simulink model "SingleInverterSim"  (R2020b)
settings: Solver=FixedStepAuto  StartTime=0.0  StopTime=3  FixedStep=Ts  RelTol=1e-3
values from neighbouring files (symbols this model uses):
  Cf = 0.02/W    (= 6.36619772368e-05)    [CalcSwingDroop.m]    (also in SingleInverterSim_Para.m = 0.02; SingleInverterSim_Para_v2.m = 0.02)
  Lc = 0.01/W    (= 3.18309886184e-05)    [CalcSwingDroop.m]    (also in SingleInverterSim_Para.m = 1e-09; SingleInverterSim_Para_v2.m = 0.01)
  Lf = 0.05/W    (= 0.000159154943092)    [CalcSwingDroop.m]    (also in SingleInverterSim_Para.m = 0.05; SingleInverterSim_Para_v2.m = 0.05)
  m = m*Wbase    (= 15.7079632679)    [CalcSwingDroop.m]    (also in SingleInverterSim_Para.m = 0.05; SingleInverterSim_Para_v2.m = 0.05)
  R_rated_GFL = X_rated_GFL/5    (= 0.08)    [SingleInverterSim_Para.m]
  R_rated_GFM = X_rated_GFM/5    (= 0.06)    [SingleInverterSim_Para.m]
  Sbase = 1    [MainAnalysisImpedanceCircuit.m]    (also in SingleInverterSim_Para.m; SingleInverterSim_Para_v2.m)
  Scale_ki_v = 20    [SingleInverterSim_Para.m]    (also in SingleInverterSim_Para_v2.m)
  Ts = 1/Fs    (= 0.0001)    [SingleInverterSim_Para.m]    (also in SingleInverterSim_Para_v2.m)
  Vbase = 1    [MainAnalysisImpedanceCircuit.m]    (also in SingleInverterSim_Para.m; SingleInverterSim_Para_v2.m)
  w_droop = 0.1*2*pi    (= 0.628318530718)    [SingleInverterSim_Para.m]    (also in SingleInverterSim_Para_v2.m = 62.8318530718)
  w_i_GFL = 250 *2*pi    (= 1570.79632679)    [SingleInverterSim_Para.m]    (also in SingleInverterSim_Para_v2.m = 3141.59265359)
  w_i_GFM = 500*2*pi    (= 3141.59265359)    [SingleInverterSim_Para.m]    (also in SingleInverterSim_Para_v2.m)
  w_pll = 15 *2*pi    (= 94.2477796077)    [SingleInverterSim_Para.m]    (also in SingleInverterSim_Para_v2.m = 62.8318530718)
  w_tau = 1e3 *2*pi    (= 6283.18530718)    [SingleInverterSim_Para.m]    (also in SingleInverterSim_Para_v2.m)
  w_v_GFM = 250 *2*pi    (= 1570.79632679)    [SingleInverterSim_Para.m]    (also in SingleInverterSim_Para_v2.m)
  Wbase = 2*pi*50    (= 314.159265359)    [CalcSwingDroop.m]    (also in MainAnalysisImpedanceCircuit.m; SingleInverterSim_Para.m; SingleInverterSim_Para_v2.m)
  X_rated_GFL = 0.4    [SingleInverterSim_Para.m]
  X_rated_GFM = 0.3    [SingleInverterSim_Para.m]
  Zbase = Vbase/Ibase    (= 1)    [MainAnalysisImpedanceCircuit.m]    (also in SingleInverterSim_Para.m; SingleInverterSim_Para_v2.m)
undefined symbols (not defined in the file or in its folder): DiscIntNeverNeededParam, initial, magnitude
libraries: powerlib x230, SimplexPS x57, SimplexPS_2015a x10, SimplusGT x3
(part 1 of 5)
settings Model: Creator=admin_user  LastModifiedBy=admin_user
settings DataIOCC: SaveOutput=off  SignalLogging=off  DSMLogging=off  SaveTime=off  ReturnWorkspaceOutputs=off

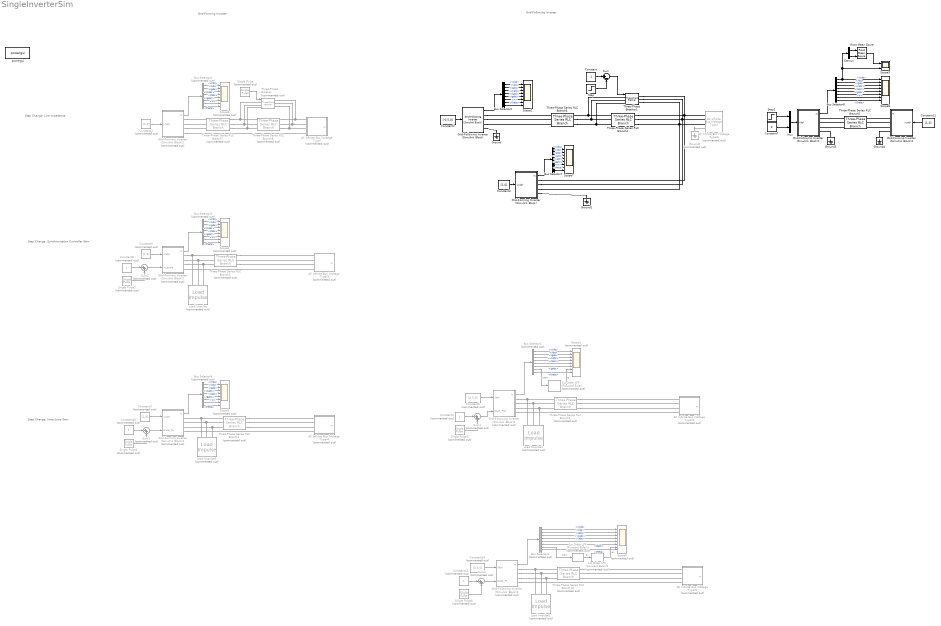
== system SingleInverterSim ==
  note: Step Change:
      | Line Impedance
  note: Grid-Forming Inverter
  note: Grid-Following Inverter
  note: Step Change:
      | Synchronization Controller Gain
  note: Step Change:
      | Inner-Loop Gain
  1st Order LPF (Forward Euler) : SimplexPS/1st Order LPF (Forward Euler)  Commented=on  wc=100*2*pi  Ts=Ts
      settings: SourceProductName=Simplex Power Systems
  1st Order LPF (Forward Euler)1 : SimplexPS/1st Order LPF (Forward Euler)  Commented=on  wc=100*2*pi  Ts=Ts
      settings: SourceProductName=Simplex Power Systems
  1st Order LPF (Forward Euler)2 : SimplexPS/1st Order LPF (Forward Euler)  Commented=on  wc=100*2*pi  Ts=Ts
      settings: SourceProductName=Simplex Power Systems
  AC Infinite Bus (Voltage Type) : Subsystem  Commented=on  AncestorBlock=|  mask{Ts=Ts, Sbase=Sbase, Vbase=Vbase, Wbase=Wbase, vd=1, vq=0, theta0=0, w=Wbase, R=1e-30}
      | SimplexPS/AC Infinite Bus
      | (Voltage Type)
      mask prompts: Ts "Ts (s), samping period"; Sbase "Sbase (VA), power base"; Vbase "Vbase (V), voltage base"; Wbase "Wbase (rad/s), frequency base"; vd "vd (pu), d-axis voltage"; vq "vq (pu), q-axis voltage"; theta0 "theta0 (rad), initial angle"; w "w (rad/s), frequency"; R "R (Ohm), resistance"
  AC Infinite Bus (Voltage Type)2 : Subsystem  Commented=on  AncestorBlock=|  mask{Ts=Ts, Sbase=Sbase, Vbase=Vbase, Wbase=Wbase, vd=1, vq=0, theta0=0, w=Wbase, R=1e-30}
      | SimplexPS/AC Infinite Bus
      | (Voltage Type)
      mask prompts: Ts "Ts (s), samping period"; Sbase "Sbase (VA), power base"; Vbase "Vbase (V), voltage base"; Wbase "Wbase (rad/s), frequency base"; vd "vd (pu), d-axis voltage"; vq "vq (pu), q-axis voltage"; theta0 "theta0 (rad), initial angle"; w "w (rad/s), frequency"; R "R (Ohm), resistance"
  AC Infinite Bus (Voltage Type)3 : Subsystem  Commented=on  AncestorBlock=|  mask{Ts=Ts, Sbase=Sbase, Vbase=Vbase, Wbase=Wbase, vd=1, vq=0, theta0=0, w=Wbase, R=1e-30}
      | SimplexPS/AC Infinite Bus
      | (Voltage Type)
      mask prompts: Ts "Ts (s), samping period"; Sbase "Sbase (VA), power base"; Vbase "Vbase (V), voltage base"; Wbase "Wbase (rad/s), frequency base"; vd "vd (pu), d-axis voltage"; vq "vq (pu), q-axis voltage"; theta0 "theta0 (rad), initial angle"; w "w (rad/s), frequency"; R "R (Ohm), resistance"
  AC Infinite Bus (Voltage Type)4 : Subsystem  Commented=on  AncestorBlock=|  mask{Ts=Ts, Sbase=Sbase, Vbase=Vbase, Wbase=Wbase, vd=1, vq=0, theta0=0, w=Wbase, R=1e-30}
      | SimplexPS/AC Infinite Bus
      | (Voltage Type)
      mask prompts: Ts "Ts (s), samping period"; Sbase "Sbase (VA), power base"; Vbase "Vbase (V), voltage base"; Wbase "Wbase (rad/s), frequency base"; vd "vd (pu), d-axis voltage"; vq "vq (pu), q-axis voltage"; theta0 "theta0 (rad), initial angle"; w "w (rad/s), frequency"; R "R (Ohm), resistance"
  AC Infinite Bus (Voltage Type)5 : Subsystem  Commented=on  AncestorBlock=|  mask{Ts=Ts, Sbase=Sbase, Vbase=Vbase, Wbase=Wbase, vd=1, vq=0, theta0=0, w=Wbase, R=1e-30}
      | SimplexPS/AC Infinite Bus
      | (Voltage Type)
      mask prompts: Ts "Ts (s), samping period"; Sbase "Sbase (VA), power base"; Vbase "Vbase (V), voltage base"; Wbase "Wbase (rad/s), frequency base"; vd "vd (pu), d-axis voltage"; vq "vq (pu), q-axis voltage"; theta0 "theta0 (rad), initial angle"; w "w (rad/s), frequency"; R "R (Ohm), resistance"
  AC Infinite Bus (Voltage Type)6 : SimplusGT/AC Infinite Bus (Voltage Type)  Commented=on  Ts=Ts  Sbase=Sbase  Vbase=Vbase  Wbase=Wbase  vd=1  vq=0  theta0=0  w=Wbase  R=1e-30
      settings: SourceProductName=Simplus Grid Tool
  Bus Selector{1,3..6} (5 alike) : BusSelector  Commented=on  OutputSignals=vcdq,ildq,igdq,vcabc,ilabc,igabc,w,theta
  Bus Selector2 : BusSelector  OutputSignals=vcdq,ildq,igdq,vcabc,ilabc,igabc,w,theta
  Bus Selector7 : BusSelector  OutputSignals=vcdq,ildq,igdq,vcabc,ilabc,igabc,w,theta
  Bus Selector8 : BusSelector  OutputSignals=vcdq,ildq,igdq,vcabc,ilabc,igabc,w,theta
  Constant : Constant
  Constant1 : Constant  Commented=on  Value=[1,0]
  Constant{4,8,10,13} (4 alike) : Constant  Commented=on
  Constant11 : Constant  Value=[1,0]
  Constant14 : Constant  Commented=on  Value=[0.5,0]
  Constant2 : Constant  Value=[-0.5,0]
  Constant3 : Constant  Value=[1,0]
  Constant5 : Constant  Commented=on  Value=[1,0]
  Constant6 : Constant  Commented=on  Value=[0.5,0]
  Constant7 : Constant  Value=0
  Constant9 : Constant  Commented=on  Value=[1,0]
  Demux : Demux  Outputs=2
  Grid-Following Inverter (Simulink Block) : SimplusGT/Grid-Following Inverter (Simulink Block)  Ts=Ts  Sbase=Sbase  Vbase=Vbase  Wbase=Wbase  w_i=w_i_GFL  w_pll=w_pll  w_tau=w_tau  Lf=Lf  Cf=Cf  Lc=Lc
      settings: SourceProductName=Simplus Grid Tool
  Grid-Following Inverter (Simulink Block)1 : Subsystem  AncestorBlock=|  mask{Ts=Ts, Sbase=Sbase, Vbase=Vbase, Wbase=Wbase, w_i=w_i_GFL, w_pll=w_pll/10, w_tau=w_tau, Lf=Lf, Cf=Cf, Lc=Lc}
      | SimplusGT/Grid-Following Inverter
      | (Simulink Block)
      mask prompts: Ts "Ts (s), sampling period"; Sbase "Sbase (VA), base power"; Vbase "Vbase (V), base voltage"; Wbase "Wbase (rad/s), base frequency"; w_i "w_i (rad/s), current-loop bandwidth"; w_pll "w_pll (rad/s), PLL bandwidth"; w_tau "w_tau (rad/s), PLL filter bandwidth"; Lf "Lf (pu), LCL filter"; Cf "Cf (pu), LCL filter"; Lc "Lc (pu), LCL filter"
  Grid-Following Inverter (Simulink Block)2 : Subsystem  Commented=on  AncestorBlock=|  mask{Ts=Ts, Sbase=Sbase, Vbase=Vbase, Wbase=Wbase, w_i=w_i_GFL, w_pll=w_pll, w_tau=w_tau, Lf=Lf, Cf=Cf, Lc=Lc}
      | SimplexPS/Grid-Following Inverter
      | (Simulink Block)
      mask prompts: Ts "Ts (s), sampling period"; Sbase "Sbase (VA), base power"; Vbase "Vbase (V), base voltage"; Wbase "Wbase (rad/s), base frequency"; w_i "w_i (rad/s), current-loop bandwidth"; w_pll "w_pll (rad/s), PLL bandwidth"; w_tau "w_tau (rad/s), PLL filter bandwidth"; Lf "Lf (pu), LCL filter"; Cf "Cf (pu), LCL filter"; Lc "Lc (pu), LCL filter"
  Grid-Following Inverter (Simulink Block)3 : Subsystem  Commented=on  AncestorBlock=|  mask{Ts=Ts, Sbase=Sbase, Vbase=Vbase, Wbase=Wbase, w_i=w_i_GFL, w_pll=w_pll, w_tau=w_tau, Lf=Lf, Cf=Cf, Lc=Lc}
      | SimplexPS/Grid-Following Inverter
      | (Simulink Block)
      mask prompts: Ts "Ts (s), sampling period"; Sbase "Sbase (VA), base power"; Vbase "Vbase (V), base voltage"; Wbase "Wbase (rad/s), base frequency"; w_i "w_i (rad/s), current-loop bandwidth"; w_pll "w_pll (rad/s), PLL bandwidth"; w_tau "w_tau (rad/s), PLL filter bandwidth"; Lf "Lf (pu), LCL filter"; Cf "Cf (pu), LCL filter"; Lc "Lc (pu), LCL filter"
  Grid-Forming Inverter (Simulink Block) : Subsystem  AncestorBlock=|  mask{Ts=Ts, Sbase=Sbase, Vbase=Vbase, Wbase=Wbase, w_i=w_i_GFM, w_v=w_v_GFM, w_droop=w_droop, m=m, Lf=Lf, Cf=Cf, Lc=Lc}
      | SimplusGT/Grid-Forming Inverter
      | (Simulink Block)
      mask prompts: Ts "Ts (s), sampling period"; Sbase "Sbase (VA), base power"; Vbase "Vbase (V), base voltage"; Wbase "Wbase (rad/s), base frequency"; w_i "w_i (rad/s), current-loop bandwidth"; w_v "w_v (rad/s), voltage-loop bandwidth"; w_droop "w_droop (rad/s), droop bandwidth"; m "m (pu), frequency droop gain"; Lf "Lf (pu), LCL filter"; Cf "Cf (pu), LCL filter"; Lc "Lc (pu), LCL filter"
  Grid-Forming Inverter (Simulink Block)1 : Subsystem  Commented=on  AncestorBlock=|  mask{Ts=Ts, Sbase=Sbase, Vbase=Vbase, Wbase=Wbase, w_i=w_i_GFM, w_v=w_v_GFM, w_droop=w_droop, m=m, Lf=Lf, Cf=Cf, Lc=Lc}
      | SimplexPS/Grid-Forming Inverter
      | (Simulink Block)
      mask prompts: Ts "Ts (s), sampling period"; Sbase "Sbase (VA), base power"; Vbase "Vbase (V), base voltage"; Wbase "Wbase (rad/s), base frequency"; w_i "w_i (rad/s), current-loop bandwidth"; w_v "w_v (rad/s), voltage-loop bandwidth"; w_droop "w_droop (rad/s), droop bandwidth"; m "m (pu), frequency droop gain"; Lf "Lf (pu), LCL filter"; Cf "Cf (pu), LCL filter"; Lc "Lc (pu), LCL filter"
  Grid-Forming Inverter (Simulink Block)2 : Subsystem  Commented=on  AncestorBlock=|  mask{Ts=Ts, Sbase=Sbase, Vbase=Vbase, Wbase=Wbase, w_i=w_i_GFM, w_v=w_v_GFM, w_droop=w_droop, m=m, Lf=Lf, Cf=Cf, Lc=Lc, Scale_ki_v=Scale_ki_v}
      | SimplexPS/Grid-Forming Inverter
      | (Simulink Block)
      mask prompts: Ts "Ts (s), sampling period"; Sbase "Sbase (VA), base power"; Vbase "Vbase (V), base voltage"; Wbase "Wbase (rad/s), base frequency"; w_i "w_i (rad/s), current-loop bandwidth"; w_v "w_v (rad/s), voltage-loop bandwidth"; w_droop "w_droop (rad/s), droop bandwidth"; m "m (pu), frequency droop gain"; Lf "Lf (pu), LCL filter"; Cf "Cf (pu), LCL filter"; Lc "Lc (pu), LCL filter"
  Grid-Forming Inverter (Simulink Block)3 : Subsystem  Commented=on  AncestorBlock=|  mask{Ts=Ts, Sbase=Sbase, Vbase=Vbase, Wbase=Wbase, w_i=w_i_GFM, w_v=w_v_GFM, w_droop=w_droop, m=m, Lf=Lf, Cf=Cf, Lc=Lc, Scale_ki_v=Scale_ki_v}
      | SimplexPS/Grid-Forming Inverter
      | (Simulink Block)
      mask prompts: Ts "Ts (s), sampling period"; Sbase "Sbase (VA), base power"; Vbase "Vbase (V), base voltage"; Wbase "Wbase (rad/s), base frequency"; w_i "w_i (rad/s), current-loop bandwidth"; w_v "w_v (rad/s), voltage-loop bandwidth"; w_droop "w_droop (rad/s), droop bandwidth"; m "m (pu), frequency droop gain"; Lf "Lf (pu), LCL filter"; Cf "Cf (pu), LCL filter"; Lc "Lc (pu), LCL filter"
  Grid-Forming Inverter (Simulink Block)4 : Subsystem  AncestorBlock=|  mask{Ts=Ts, Sbase=Sbase, Vbase=Vbase, Wbase=Wbase, w_i=w_i_GFM, w_v=w_v_GFM, w_droop=w_droop*100, m=m, Lf=Lf, Cf=Cf, Lc=Lc}
      | SimplusGT/Grid-Forming Inverter
      | (Simulink Block)
      mask prompts: Ts "Ts (s), sampling period"; Sbase "Sbase (VA), base power"; Vbase "Vbase (V), base voltage"; Wbase "Wbase (rad/s), base frequency"; w_i "w_i (rad/s), current-loop bandwidth"; w_v "w_v (rad/s), voltage-loop bandwidth"; w_droop "w_droop (rad/s), droop bandwidth"; m "m (pu), frequency droop gain"; Lf "Lf (pu), LCL filter"; Cf "Cf (pu), LCL filter"; Lc "Lc (pu), LCL filter"
  Ground{,1,3..4} (4 alike) : powerlib/Elements/Ground  LConnTagsString=a
  Ground2 : powerlib/Elements/Ground  Commented=on  LConnTagsString=a
  Load Impulse{,1..3} (4 alike) : SimplexPS/Load Impulse  Commented=on  t0=t0  dt=Ts  R=10000*Zbase
      settings: SourceProductName=Simplex Power Systems
  Mux : Mux  Inputs=2
  Root Mean Squre : SimplusGT/Root Mean Squre  SystemSampleTime=-1  VariantActivationTime=update diagram  Latency=0  AutoFrameSizeCalculation=off
      settings: SourceProductName=Simplus Grid Tool
  Scope{1,3..6} (5 alike) : Scope  Commented=on  NumInputPorts=8
  Scope2 : Scope  NumInputPorts=8
  Scope7 : Scope  NumInputPorts=8
  Scope8 : Scope  NumInputPorts=8
  Scope9 : Scope  NumInputPorts=2
  Single Pulse : SimplexPS/Single Pulse  Commented=on  t0=t0  dt=dt  Am=1
      settings: SourceProductName=Simplex Power Systems
  Single Pulse2 : SimplexPS/Single Pulse  Commented=on  t0=t0  dt=dt  Am=3
      settings: SourceProductName=Simplex Power Systems
  Single Pulse3 : SimplexPS/Single Pulse  Commented=on  t0=2  dt=0.2  Am=3
      settings: SourceProductName=Simplex Power Systems
  Single Pulse4 : SimplexPS/Single Pulse  Commented=on  t0=t0  dt=dt  Am=-2/5
      settings: SourceProductName=Simplex Power Systems
  Single Pulse5 : SimplexPS/Single Pulse  Commented=on  t0=t0  dt=dt  Am=-2/5
      settings: SourceProductName=Simplex Power Systems
  Step : Step  SampleTime=0
  Step1 : Step  After=0.5  SampleTime=0
  Sum : Sum  Inputs=|+-
  Sum{1..4} (4 alike) : Sum  Commented=on  Inputs=|++
  Three-Phase Series RLC Branch1 : powerlib/Elements/Three-Phase Series RLC Branch  Commented=on  LConnTagsString=A|B|C  RConnTagsString=A|B|C  BranchType=RL  Resistance=R_rated_GFM*Zbase  Inductance=X_rated_GFM*Zbase/Wbase  Capacitance=1/Wbase  Measurements=None
  Three-Phase Series RLC Branch10 : powerlib/Elements/Three-Phase Series RLC Branch  Commented=on  LConnTagsString=A|B|C  RConnTagsString=A|B|C  BranchType=RL  Resistance=R_rated_GFL*Zbase  Inductance=X_rated_GFL*Zbase/Wbase  Capacitance=1/Wbase  Measurements=None
  Three-Phase Series RLC Branch2 : powerlib/Elements/Three-Phase Series RLC Branch  Commented=on  LConnTagsString=A|B|C  RConnTagsString=A|B|C  BranchType=RL  Resistance=R_rated_GFL*Zbase  Inductance=X_rated_GFL*Zbase/Wbase  Capacitance=1/Wbase  Measurements=None
  Three-Phase Series RLC Branch3 : powerlib/Elements/Three-Phase Series RLC Branch  Commented=on  LConnTagsString=A|B|C  RConnTagsString=A|B|C  BranchType=RL  Resistance=R_rated_GFM*Zbase  Inductance=X_rated_GFM*Zbase/Wbase  Capacitance=1/Wbase  Measurements=None
  Three-Phase Series RLC Branch4 : powerlib/Elements/Three-Phase Series RLC Branch  LConnTagsString=A|B|C  RConnTagsString=A|B|C  BranchType=RL  Resistance=0.23*Zbase/10  Inductance=0.23*Zbase/Wbase  Capacitance=1/Wbase  Measurements=None
  Three-Phase Series RLC Branch5 : powerlib/Elements/Three-Phase Series RLC Branch  LConnTagsString=A|B|C  RConnTagsString=A|B|C  BranchType=RL  Resistance=0.1*Zbase/10  Inductance=0.1*Zbase/Wbase  Capacitance=1/Wbase  Measurements=None
  Three-Phase Series RLC Branch6 : powerlib/Elements/Three-Phase Series RLC Branch  LConnTagsString=A|B|C  RConnTagsString=A|B|C  BranchType=RL  Resistance=0.3*Zbase/10  Inductance=0.3*Zbase/Wbase  Capacitance=1/Wbase  Measurements=None
  Three-Phase Series RLC Branch7 : powerlib/Elements/Three-Phase Series RLC Branch  Commented=on  LConnTagsString=A|B|C  RConnTagsString=A|B|C  BranchType=RL  Resistance=0.1*Zbase/5  Inductance=0.1*Zbase/Wbase  Capacitance=1/Wbase  Measurements=None
  Three-Phase Series RLC Branch8 : powerlib/Elements/Three-Phase Series RLC Branch  Commented=on  LConnTagsString=A|B|C  RConnTagsString=A|B|C  BranchType=RL  Resistance=0.2*Zbase/5  Inductance=0.2*Zbase/Wbase  Capacitance=1/Wbase  Measurements=None
  Three-Phase Breaker : powerlib/Elements/Three-Phase Breaker  Commented=on  InitialState=open  SwitchA=on  SwitchB=on  SwitchC=on  SwitchTimes="[1/60  5/60]"  External=on  BreakerResistance=0.01  SnubberResistance=1e6  SnubberCapacitance=inf  Measurements=None
  Three-Phase Breaker1 : powerlib/Elements/Three-Phase Breaker  InitialState=open  SwitchA=on  SwitchB=on  SwitchC=on  SwitchTimes="[1/60  5/60]"  External=on  BreakerResistance=0.01  SnubberResistance=1e6  SnubberCapacitance=inf  Measurements=None
  powergui : powerlib/powergui  Priority=1  SimulationMode=Discrete  SampleTime=Ts  frequency=60  Iterations=50  frequencyindice=0  Pbase=100e6  ErrMax=1e-4  UnitsV=kV  UnitsW=MW  buscounter=0  FunctionMessages=off  echomessages=off  EnableUseOfTLC=off  CurrentSourceSwitches=off  DisableSnubberDevices=off  DisableRonSwitches=off  DisableVfSwitches=off  DisplayEquations=off  AutomaticDiscreteSolvers=off  SolverType=Tustin/Backward Euler (TBE)  Interpol=off  ExternalGateDelay=off  methode=off  Ts=100  x0status=blocks  SPID=on  SwTol=0  HookPort=off  NonlinearTolerance=1e-4  nMaxIteration=100  ContinueOnMaxIteration=off  RestoreLinks=warning  ResistiveCurrentMeasurement=off  Frange=[0:2:500]  Ylog=off  Xlog=on  ShowGrid=off  save=off  variable=ZData  structure=0  ZoomFFT=off  StartTime=0.0  cycles=1  DisplayStyle=1  fundamental=60  FreqAxis=off  MaxFrequency=1000  frequencyindicesteady=1  RmsSteady=1  display=off
  wires:
  Bus Selector2/7 -> Scope2/7  "<w>"
  Bus Selector2/5 -> Scope2/5  "<ilabc>"
  Bus Selector2/6 -> Scope2/6  "<igabc>"
  Bus Selector2/3 -> Scope2/3  "<igdq>"
  Bus Selector2/8 -> Scope2/8  "<theta>"
  Bus Selector2/4 -> Scope2/4  "<vcabc>"
  Bus Selector2/1 -> Scope2/1  "<vcdq>"
  Bus Selector2/2 -> Scope2/2  "<ildq>"
  Grid-Following Inverter (Simulink Block)/1 -> Bus Selector2/1
  Bus Selector4/4 -> Scope3/4  "<vcabc>"
  Grid-Forming Inverter (Simulink Block)1/1(m) -> Bus Selector4/1
  Bus Selector4/3 -> Scope3/3  "<igdq>"
  Bus Selector4/2 -> Scope3/2  "<ildq>"
  Bus Selector4/1 -> Scope3/1  "<vcdq>"
  Bus Selector4/5 -> Scope3/5  "<ilabc>"
  Bus Selector4/6 -> Scope3/6  "<igabc>"
  Bus Selector4/7 -> Scope3/7  "<w>"
  Bus Selector4/8 -> Scope3/8  "<theta>"
  Constant1/1 -> Grid-Forming Inverter (Simulink Block)1/1(vcdq*)
  Single Pulse/1 -> Three-Phase Breaker/1
  Constant/1 -> Sum/1
  Step/1 -> Sum/2
  Sum/1 -> Three-Phase Breaker1/1
  Grid-Following Inverter (Simulink Block)2/1(m) -> Bus Selector1/1
  Constant5/1 -> Grid-Forming Inverter (Simulink Block)2/1(vcdq*)
  Grid-Forming Inverter (Simulink Block)2/1(m) -> Bus Selector3/1
  Bus Selector3/8 -> Scope4/8  "<theta>"
  Bus Selector1/5 -> Scope1/5  "<ilabc>"
  Bus Selector3/2 -> Scope4/2  "<ildq>"
  Bus Selector3/1 -> Scope4/1  "<vcdq>"
  Bus Selector3/7 -> Scope4/7  "<w>"
  Bus Selector3/3 -> Scope4/3  "<igdq>"
  Bus Selector3/4 -> Scope4/4  "<vcabc>"
  Bus Selector1/6 -> Scope1/6  "<igabc>"
  Bus Selector1/3 -> Scope1/3  "<igdq>"
  Bus Selector3/6 -> Scope4/6  "<igabc>"
  Bus Selector1/8 -> Scope1/8  "<theta>"
  Bus Selector1/1 -> Scope1/1  "<vcdq>"
  Bus Selector1/4 -> Scope1/4  "<vcabc>"
  Bus Selector1/2 -> Scope1/2  "<ildq>"
  Bus Selector3/5 -> Scope4/5  "<ilabc>"
  Sum2/1 -> Grid-Forming Inverter (Simulink Block)2/2(m_scale)
  Constant8/1 -> Sum2/1
  Single Pulse2/1 -> Sum2/2
  Constant4/1 -> Sum1/1
  Sum1/1 -> Grid-Following Inverter (Simulink Block)2/2(Scale_PIpll)
  Single Pulse3/1 -> Sum1/2
  Bus Selector1/7 -> 1st Order LPF (Forward Euler)/1  "<w>"
  1st Order LPF (Forward Euler)/1 -> Scope1/7  "w"
  Constant9/1 -> Grid-Forming Inverter (Simulink Block)3/1(vcdq*)
  Grid-Forming Inverter (Simulink Block)3/1(m) -> Bus Selector5/1
  Bus Selector5/8 -> Scope5/8  "<theta>"
  Bus Selector5/2 -> Scope5/2  "<ildq>"
  Bus Selector5/1 -> Scope5/1  "<vcdq>"
  Bus Selector5/7 -> Scope5/7  "<w>"
  Bus Selector5/4 -> Scope5/4  "<vcabc>"
  Bus Selector5/3 -> Scope5/3  "<igdq>"
  Bus Selector5/5 -> Scope5/5  "<ilabc>"
  Bus Selector5/6 -> Scope5/6  "<igabc>"
  Grid-Following Inverter (Simulink Block)3/1(m) -> Bus Selector6/1
  Bus Selector6/5 -> Scope6/5  "<ilabc>"
  Bus Selector6/6 -> Scope6/6  "<igabc>"
  Bus Selector6/3 -> Scope6/3  "<igdq>"
  Bus Selector6/8 -> Scope6/8  "<theta>"
  Bus Selector6/1 -> Scope6/1  "<vcdq>"
  Bus Selector6/4 -> Scope6/4  "<vcabc>"
  Bus Selector6/2 -> Scope6/2  "<ildq>"
  Constant10/1 -> Sum3/1
  Sum3/1 -> Grid-Forming Inverter (Simulink Block)3/2(Scale_PIv)
  Sum4/1 -> Grid-Following Inverter (Simulink Block)3/2(Scale_PIi)
  Single Pulse5/1 -> Sum4/2
  Constant13/1 -> Sum4/1
  Single Pulse4/1 -> Sum3/2
  1st Order LPF (Forward Euler)1/1 -> Scope6/7  "w"
  1st Order LPF (Forward Euler)2/1 -> 1st Order LPF (Forward Euler)1/1  "w"
  Bus Selector6/7 -> 1st Order LPF (Forward Euler)2/1  "<w>"
  Constant14/1 -> Grid-Following Inverter (Simulink Block)3/1(ildq*)
  Constant6/1 -> Grid-Following Inverter (Simulink Block)2/1(ildq*)
  Constant2/1 -> Grid-Following Inverter (Simulink Block)/1
  Constant3/1 -> Grid-Forming Inverter (Simulink Block)/1(vcdq*)
  Grid-Forming Inverter (Simulink Block)/1(m) -> Bus Selector7/1
  Bus Selector7/1 -> Scope7/1  "<vcdq>"
  Bus Selector7/2 -> Scope7/2  "<ildq>"
  Bus Selector7/3 -> Scope7/3  "<igdq>"
  Bus Selector7/4 -> Scope7/4  "<vcabc>"
  Bus Selector7/5 -> Scope7/5  "<ilabc>"
  Bus Selector7/7 -> Scope7/7  "<w>"
  Bus Selector7/6 -> Scope7/6  "<igabc>"
  Bus Selector7/8 -> Scope7/8  "<theta>"
  Grid-Following Inverter (Simulink Block)1/1(m) -> Bus Selector8/1
  Bus Selector8/1 -> Demux/1, Scope9/2, Scope8/1  "<vcdq>"
  Bus Selector8/2 -> Scope8/2  "<ildq>"
  Bus Selector8/3 -> Scope8/3  "<igdq>"
  Bus Selector8/4 -> Scope8/4  "<vcabc>"
  Bus Selector8/5 -> Scope8/5  "<ilabc>"
  Bus Selector8/6 -> Scope8/6  "<igabc>"
  Bus Selector8/7 -> Scope8/7  "<w>"
  Bus Selector8/8 -> Scope8/8  "<theta>"
  Mux/1 -> Grid-Following Inverter (Simulink Block)1/1(ildq*)
  Constant7/1 -> Mux/2
  Step1/1 -> Mux/1
  Constant11/1 -> Grid-Forming Inverter (Simulink Block)4/1(vcdq*)
  Demux/2 -> Root Mean Squre/2
  Demux/1 -> Root Mean Squre/1
  Root Mean Squre/1 -> Scope9/1
  connections:
  Grid-Following Inverter (Simulink Block)/RConn1 -- Three-Phase Series RLC Branch6/RConn1
  Grid-Following Inverter (Simulink Block)/RConn2 -- Three-Phase Series RLC Branch6/RConn2
  Grid-Following Inverter (Simulink Block)/RConn3 -- Three-Phase Series RLC Branch6/RConn3
  Grid-Forming Inverter (Simulink Block)1/RConn1 -- Three-Phase Series RLC Branch7/RConn1
  Grid-Forming Inverter (Simulink Block)1/RConn2 -- Three-Phase Series RLC Branch7/RConn2
  Grid-Forming Inverter (Simulink Block)1/RConn3 -- Three-Phase Series RLC Branch7/RConn3
  Grid-Forming Inverter (Simulink Block)1/RConn4 -- AC Infinite Bus (Voltage Type)/LConn4
  Three-Phase Series RLC Branch7/LConn1 -- Three-Phase Breaker/LConn1 -- Three-Phase Series RLC Branch8/RConn1
  Three-Phase Series RLC Branch7/LConn2 -- Three-Phase Breaker/LConn2 -- Three-Phase Series RLC Branch8/RConn2
  Three-Phase Series RLC Branch7/LConn3 -- Three-Phase Breaker/LConn3 -- Three-Phase Series RLC Branch8/RConn3
  Three-Phase Series RLC Branch8/LConn1 -- Three-Phase Breaker/RConn1 -- AC Infinite Bus (Voltage Type)/LConn1
  Three-Phase Series RLC Branch8/LConn2 -- AC Infinite Bus (Voltage Type)/LConn2 -- Three-Phase Breaker/RConn2
  Three-Phase Series RLC Branch8/LConn3 -- AC Infinite Bus (Voltage Type)/LConn3 -- Three-Phase Breaker/RConn3
  Three-Phase Series RLC Branch4/RConn1 -- Three-Phase Breaker1/LConn1 -- Three-Phase Series RLC Branch6/LConn1
  Three-Phase Series RLC Branch6/LConn2 -- Three-Phase Breaker1/LConn2 -- Three-Phase Series RLC Branch4/RConn2
  Three-Phase Series RLC Branch6/LConn3 -- Three-Phase Breaker1/LConn3 -- Three-Phase Series RLC Branch4/RConn3
  Three-Phase Series RLC Branch4/LConn1 -- Grid-Forming Inverter (Simulink Block)/RConn1 -- AC Infinite Bus (Voltage Type)6/LConn1 -- Three-Phase Breaker1/RConn1
  Three-Phase Series RLC Branch4/LConn2 -- Grid-Forming Inverter (Simulink Block)/RConn2 -- AC Infinite Bus (Voltage Type)6/LConn2 -- Three-Phase Breaker1/RConn2
  Three-Phase Series RLC Branch4/LConn3 -- Grid-Forming Inverter (Simulink Block)/RConn3 -- AC Infinite Bus (Voltage Type)6/LConn3 -- Three-Phase Breaker1/RConn3
  Grid-Following Inverter (Simulink Block)2/RConn1 -- Load Impulse1/LConn1 -- Three-Phase Series RLC Branch2/RConn1
  Grid-Following Inverter (Simulink Block)2/RConn2 -- Load Impulse1/LConn2 -- Three-Phase Series RLC Branch2/RConn2
  Grid-Forming Inverter (Simulink Block)2/RConn2 -- Load Impulse/LConn2 -- Three-Phase Series RLC Branch3/RConn2
  Grid-Following Inverter (Simulink Block)2/RConn3 -- Load Impulse1/LConn3 -- Three-Phase Series RLC Branch2/RConn3
  Grid-Forming Inverter (Simulink Block)2/RConn3 -- Load Impulse/LConn3 -- Three-Phase Series RLC Branch3/RConn3
  Grid-Forming Inverter (Simulink Block)2/RConn1 -- Load Impulse/LConn1 -- Three-Phase Series RLC Branch3/RConn1
  Grid-Following Inverter (Simulink Block)2/RConn4 -- AC Infinite Bus (Voltage Type)3/LConn4
  AC Infinite Bus (Voltage Type)2/LConn4 -- Grid-Forming Inverter (Simulink Block)2/RConn4
  Three-Phase Series RLC Branch3/LConn1 -- AC Infinite Bus (Voltage Type)2/LConn1
  AC Infinite Bus (Voltage Type)2/LConn2 -- Three-Phase Series RLC Branch3/LConn2
  Three-Phase Series RLC Branch3/LConn3 -- AC Infinite Bus (Voltage Type)2/LConn3
  Three-Phase Series RLC Branch2/LConn1 -- AC Infinite Bus (Voltage Type)3/LConn1
  Three-Phase Series RLC Branch2/LConn2 -- AC Infinite Bus (Voltage Type)3/LConn2
  Three-Phase Series RLC Branch2/LConn3 -- AC Infinite Bus (Voltage Type)3/LConn3
  Grid-Forming Inverter (Simulink Block)3/RConn4 -- AC Infinite Bus (Voltage Type)4/LConn4
  Three-Phase Series RLC Branch1/RConn2 -- Load Impulse3/LConn2 -- Grid-Forming Inverter (Simulink Block)3/RConn2
  Three-Phase Series RLC Branch1/RConn1 -- Load Impulse3/LConn1 -- Grid-Forming Inverter (Simulink Block)3/RConn1
  Three-Phase Series RLC Branch1/RConn3 -- Load Impulse3/LConn3 -- Grid-Forming Inverter (Simulink Block)3/RConn3
  Grid-Following Inverter (Simulink Block)3/RConn4 -- AC Infinite Bus (Voltage Type)5/LConn4
  Grid-Following Inverter (Simulink Block)3/RConn1 -- Load Impulse2/LConn1 -- Three-Phase Series RLC Branch10/RConn1
  Grid-Following Inverter (Simulink Block)3/RConn2 -- Load Impulse2/LConn2 -- Three-Phase Series RLC Branch10/RConn2
  Grid-Following Inverter (Simulink Block)3/RConn3 -- Load Impulse2/LConn3 -- Three-Phase Series RLC Branch10/RConn3
  Three-Phase Series RLC Branch1/LConn1 -- AC Infinite Bus (Voltage Type)4/LConn1
  Three-Phase Series RLC Branch1/LConn2 -- AC Infinite Bus (Voltage Type)4/LConn2
  Three-Phase Series RLC Branch1/LConn3 -- AC Infinite Bus (Voltage Type)4/LConn3
  Three-Phase Series RLC Branch10/LConn1 -- AC Infinite Bus (Voltage Type)5/LConn1
  AC Infinite Bus (Voltage Type)5/LConn2 -- Three-Phase Series RLC Branch10/LConn2
  Three-Phase Series RLC Branch10/LConn3 -- AC Infinite Bus (Voltage Type)5/LConn3
  Grid-Following Inverter (Simulink Block)/RConn4 -- Ground/LConn1
  Grid-Forming Inverter (Simulink Block)/RConn4 -- Ground1/LConn1
  Ground2/LConn1 -- AC Infinite Bus (Voltage Type)6/LConn4
  Three-Phase Series RLC Branch5/RConn1 -- Grid-Following Inverter (Simulink Block)1/RConn1
  Three-Phase Series RLC Branch5/RConn3 -- Grid-Following Inverter (Simulink Block)1/RConn3
  Three-Phase Series RLC Branch5/RConn2 -- Grid-Following Inverter (Simulink Block)1/RConn2
  Grid-Forming Inverter (Simulink Block)4/RConn1 -- Three-Phase Series RLC Branch5/LConn1
  Grid-Forming Inverter (Simulink Block)4/RConn2 -- Three-Phase Series RLC Branch5/LConn2
  Grid-Forming Inverter (Simulink Block)4/RConn3 -- Three-Phase Series RLC Branch5/LConn3
  Ground3/LConn1 -- Grid-Following Inverter (Simulink Block)1/RConn4
  Ground4/LConn1 -- Grid-Forming Inverter (Simulink Block)4/RConn4

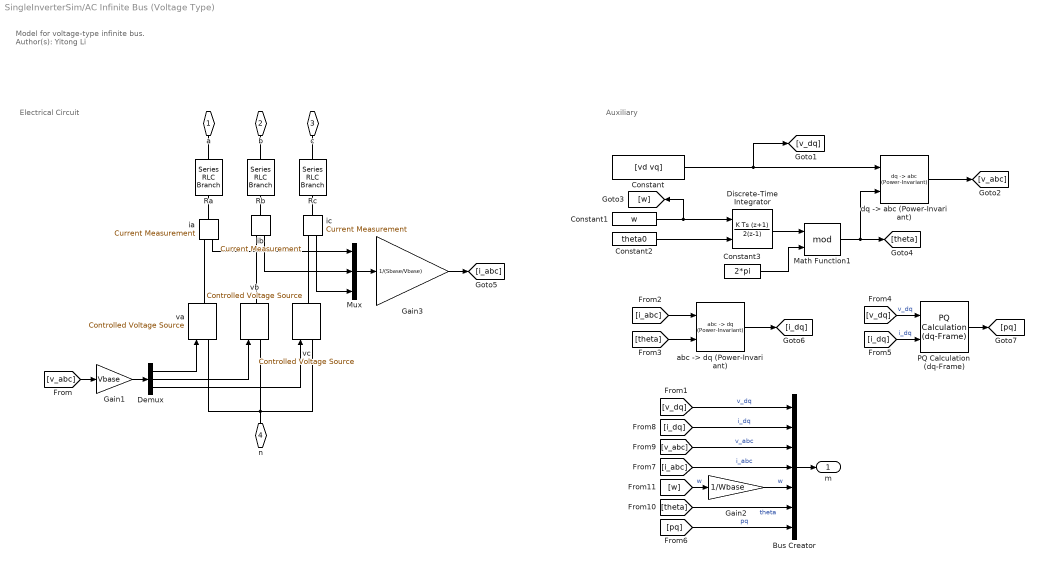
== system SingleInverterSim/AC Infinite Bus (Voltage Type) ==
  note: Model for voltage-type infinite bus.
      |
      | Author(s): Yitong Li
  note: Electrical Circuit
  note: Auxiliary
  Bus Creator : BusCreator  Inputs=7
  Constant : Constant  Value=[vd vq]
  Constant1 : Constant  Value=w
  Constant2 : Constant  Value=theta0
  Constant3 : Constant  Value=2*pi
  Demux : Demux  Outputs=3
  Discrete-Time Integrator : DiscreteIntegrator  IntegratorMethod=Integration: Trapezoidal  InitialConditionSource=external  SampleTime=-1  ICPrevOutput=DiscIntNeverNeededParam  ICPrevScaledInput=DiscIntNeverNeededParam
  Gain1 : Gain  Gain=Vbase
  Gain2 : Gain  Gain=1/Wbase
  Gain3 : Gain  Gain=1/(Sbase/Vbase)
  Math Function1 : Math  Operator=mod  SignedPower=on  SaturateOnIntegerOverflow=on
  Mux : Mux  Inputs=3
  PQ Calculation (dq-Frame) : SimplexPS/PQ Calculation (dq-Frame)  SystemSampleTime=-1  VariantActivationTime=update diagram  Latency=0  AutoFrameSizeCalculation=off
      settings: SourceProductName=Simplex Power Systems
  Ra : powerlib/Elements/Series RLC Branch  LConnTagsString=__new0  RConnTagsString=__new0  BranchType=R  Resistance=R  Inductance=1e-3  SetiL0=off  InitialCurrent=0  Capacitance=1e-6  Setx0=off  InitialVoltage=0  Measurements=None
  Rb : powerlib/Elements/Series RLC Branch  LConnTagsString=__new0  RConnTagsString=__new0  BranchType=R  Resistance=R  Inductance=1e-3  SetiL0=off  InitialCurrent=0  Capacitance=1e-6  Setx0=off  InitialVoltage=0  Measurements=None
  Rc : powerlib/Elements/Series RLC Branch  LConnTagsString=__new0  RConnTagsString=__new0  BranchType=R  Resistance=R  Inductance=1e-3  SetiL0=off  InitialCurrent=0  Capacitance=1e-6  Setx0=off  InitialVoltage=0  Measurements=None
  "abc -> dq (Power-Invariant)" : SimplexPS/abc -> dq (Power-Invariant)  SystemSampleTime=-1  VariantActivationTime=update diagram  Latency=0  AutoFrameSizeCalculation=off
      settings: SourceProductName=Simplex Power Systems
  "dq -> abc (Power-Invariant)" : SimplexPS/dq -> abc (Power-Invariant)  SystemSampleTime=-1  VariantActivationTime=update diagram  Latency=0  AutoFrameSizeCalculation=off
      settings: SourceProductName=Simplex Power Systems
  ia : powerlib/Measurements/Current Measurement  PhasorSimulation=off  OutputType=Complex  PSBequivalent=0
  ib : powerlib/Measurements/Current Measurement  PhasorSimulation=off  OutputType=Complex  PSBequivalent=0
  ic : powerlib/Measurements/Current Measurement  PhasorSimulation=off  OutputType=Complex  PSBequivalent=0
  va : powerlib/Electrical Sources/Controlled Voltage Source  Initialize=on  Source_Type=AC  Amplitude=0  Phase=0  Frequency=0  Measurements=None
  vb : powerlib/Electrical Sources/Controlled Voltage Source  Initialize=on  Source_Type=AC  Amplitude=0  Phase=0  Frequency=0  Measurements=None
  vc : powerlib/Electrical Sources/Controlled Voltage Source  Initialize=on  Source_Type=AC  Amplitude=0  Phase=0  Frequency=0  Measurements=None
  a : PMIOPort  Side=Left
  b : PMIOPort  Port=2  Side=Left
  c : PMIOPort  Port=3  Side=Left
  n : PMIOPort  Port=4  Side=Left
  m : Outport
  wires:
  [v_abc] -> Gain1/1
  Demux/1 -> va/1
  Demux/2 -> vb/1
  Demux/3 -> vc/1
  Math Function1/1 -> "dq -> abc (Power-Invariant)"/2, [theta]
  Constant2/1 -> Discrete-Time Integrator/2
  Constant1/1 -> Discrete-Time Integrator/1, [w]
  "dq -> abc (Power-Invariant)"/1 -> [v_abc]
  Constant3/1 -> Math Function1/2
  Constant/1 -> "dq -> abc (Power-Invariant)"/1, [v_dq]
  Discrete-Time Integrator/1 -> Math Function1/1
  [v_dq] -> Bus Creator/1  "v_dq"
  [i_abc] -> Bus Creator/4  "i_abc"
  [w] -> Gain2/1  "w"
  [v_abc] -> Bus Creator/3  "v_abc"
  Gain2/1 -> Bus Creator/5  "w"
  [i_dq] -> Bus Creator/2  "i_dq"
  Bus Creator/1 -> m/1
  [theta] -> Bus Creator/6  "theta"
  ia/1 -> Mux/1
  ib/1 -> Mux/2
  ic/1 -> Mux/3
  [i_abc] -> "abc -> dq (Power-Invariant)"/1
  [theta] -> "abc -> dq (Power-Invariant)"/2
  "abc -> dq (Power-Invariant)"/1 -> [i_dq]
  Gain1/1 -> Demux/1
  Mux/1 -> Gain3/1
  Gain3/1 -> [i_abc]
  [v_dq] -> PQ Calculation (dq-Frame)/1  "v_dq"
  [i_dq] -> PQ Calculation (dq-Frame)/2  "i_dq"
  PQ Calculation (dq-Frame)/1 -> [pq]
  [pq] -> Bus Creator/7  "pq"
  connections:
  vc/LConn1 -- n/RConn1 -- va/LConn1 -- vb/LConn1
  ia/RConn1 -- va/RConn1
  ib/RConn1 -- vb/RConn1
  ic/RConn1 -- vc/RConn1
  Ra/RConn1 -- ia/LConn1
  Ra/LConn1 -- a/RConn1
  ib/LConn1 -- Rb/RConn1
  Rb/LConn1 -- b/RConn1
  Rc/RConn1 -- ic/LConn1
  Rc/LConn1 -- c/RConn1

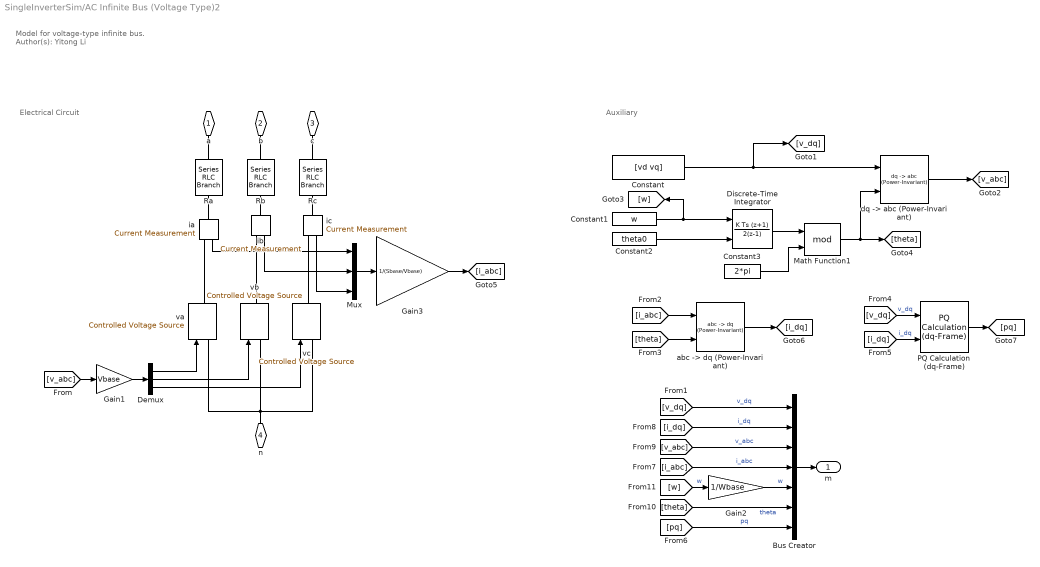
== system SingleInverterSim/AC Infinite Bus (Voltage Type)2 ==
  note: Model for voltage-type infinite bus.
      |
      | Author(s): Yitong Li
  note: Electrical Circuit
  note: Auxiliary
  Bus Creator : BusCreator  Inputs=7
  Constant : Constant  Value=[vd vq]
  Constant1 : Constant  Value=w
  Constant2 : Constant  Value=theta0
  Constant3 : Constant  Value=2*pi
  Demux : Demux  Outputs=3
  Discrete-Time Integrator : DiscreteIntegrator  IntegratorMethod=Integration: Trapezoidal  InitialConditionSource=external  SampleTime=-1  ICPrevOutput=DiscIntNeverNeededParam  ICPrevScaledInput=DiscIntNeverNeededParam
  Gain1 : Gain  Gain=Vbase
  Gain2 : Gain  Gain=1/Wbase
  Gain3 : Gain  Gain=1/(Sbase/Vbase)
  Math Function1 : Math  Operator=mod  SignedPower=on  SaturateOnIntegerOverflow=on
  Mux : Mux  Inputs=3
  PQ Calculation (dq-Frame) : SimplexPS/PQ Calculation (dq-Frame)  SystemSampleTime=-1  VariantActivationTime=update diagram  Latency=0  AutoFrameSizeCalculation=off
      settings: SourceProductName=Simplex Power Systems
  Ra : powerlib/Elements/Series RLC Branch  LConnTagsString=__new0  RConnTagsString=__new0  BranchType=R  Resistance=R  Inductance=1e-3  SetiL0=off  InitialCurrent=0  Capacitance=1e-6  Setx0=off  InitialVoltage=0  Measurements=None
  Rb : powerlib/Elements/Series RLC Branch  LConnTagsString=__new0  RConnTagsString=__new0  BranchType=R  Resistance=R  Inductance=1e-3  SetiL0=off  InitialCurrent=0  Capacitance=1e-6  Setx0=off  InitialVoltage=0  Measurements=None
  Rc : powerlib/Elements/Series RLC Branch  LConnTagsString=__new0  RConnTagsString=__new0  BranchType=R  Resistance=R  Inductance=1e-3  SetiL0=off  InitialCurrent=0  Capacitance=1e-6  Setx0=off  InitialVoltage=0  Measurements=None
  "abc -> dq (Power-Invariant)" : SimplexPS/abc -> dq (Power-Invariant)  SystemSampleTime=-1  VariantActivationTime=update diagram  Latency=0  AutoFrameSizeCalculation=off
      settings: SourceProductName=Simplex Power Systems
  "dq -> abc (Power-Invariant)" : SimplexPS/dq -> abc (Power-Invariant)  SystemSampleTime=-1  VariantActivationTime=update diagram  Latency=0  AutoFrameSizeCalculation=off
      settings: SourceProductName=Simplex Power Systems
  ia : powerlib/Measurements/Current Measurement  PhasorSimulation=off  OutputType=Complex  PSBequivalent=0
  ib : powerlib/Measurements/Current Measurement  PhasorSimulation=off  OutputType=Complex  PSBequivalent=0
  ic : powerlib/Measurements/Current Measurement  PhasorSimulation=off  OutputType=Complex  PSBequivalent=0
  va : powerlib/Electrical Sources/Controlled Voltage Source  Initialize=on  Source_Type=AC  Amplitude=0  Phase=0  Frequency=0  Measurements=None
  vb : powerlib/Electrical Sources/Controlled Voltage Source  Initialize=on  Source_Type=AC  Amplitude=0  Phase=0  Frequency=0  Measurements=None
  vc : powerlib/Electrical Sources/Controlled Voltage Source  Initialize=on  Source_Type=AC  Amplitude=0  Phase=0  Frequency=0  Measurements=None
  a : PMIOPort  Side=Left
  b : PMIOPort  Port=2  Side=Left
  c : PMIOPort  Port=3  Side=Left
  n : PMIOPort  Port=4  Side=Left
  m : Outport
  wires:
  [v_abc] -> Gain1/1
  Demux/1 -> va/1
  Demux/2 -> vb/1
  Demux/3 -> vc/1
  Math Function1/1 -> "dq -> abc (Power-Invariant)"/2, [theta]
  Constant2/1 -> Discrete-Time Integrator/2
  Constant1/1 -> Discrete-Time Integrator/1, [w]
  "dq -> abc (Power-Invariant)"/1 -> [v_abc]
  Constant3/1 -> Math Function1/2
  Constant/1 -> "dq -> abc (Power-Invariant)"/1, [v_dq]
  Discrete-Time Integrator/1 -> Math Function1/1
  [v_dq] -> Bus Creator/1  "v_dq"
  [i_abc] -> Bus Creator/4  "i_abc"
  [w] -> Gain2/1  "w"
  [v_abc] -> Bus Creator/3  "v_abc"
  Gain2/1 -> Bus Creator/5  "w"
  [i_dq] -> Bus Creator/2  "i_dq"
  Bus Creator/1 -> m/1
  [theta] -> Bus Creator/6  "theta"
  ia/1 -> Mux/1
  ib/1 -> Mux/2
  ic/1 -> Mux/3
  [i_abc] -> "abc -> dq (Power-Invariant)"/1
  [theta] -> "abc -> dq (Power-Invariant)"/2
  "abc -> dq (Power-Invariant)"/1 -> [i_dq]
  Gain1/1 -> Demux/1
  Mux/1 -> Gain3/1
  Gain3/1 -> [i_abc]
  [v_dq] -> PQ Calculation (dq-Frame)/1  "v_dq"
  [i_dq] -> PQ Calculation (dq-Frame)/2  "i_dq"
  PQ Calculation (dq-Frame)/1 -> [pq]
  [pq] -> Bus Creator/7  "pq"
  connections:
  vc/LConn1 -- n/RConn1 -- va/LConn1 -- vb/LConn1
  ia/RConn1 -- va/RConn1
  ib/RConn1 -- vb/RConn1
  ic/RConn1 -- vc/RConn1
  Ra/RConn1 -- ia/LConn1
  Ra/LConn1 -- a/RConn1
  ib/LConn1 -- Rb/RConn1
  Rb/LConn1 -- b/RConn1
  Rc/RConn1 -- ic/LConn1
  Rc/LConn1 -- c/RConn1

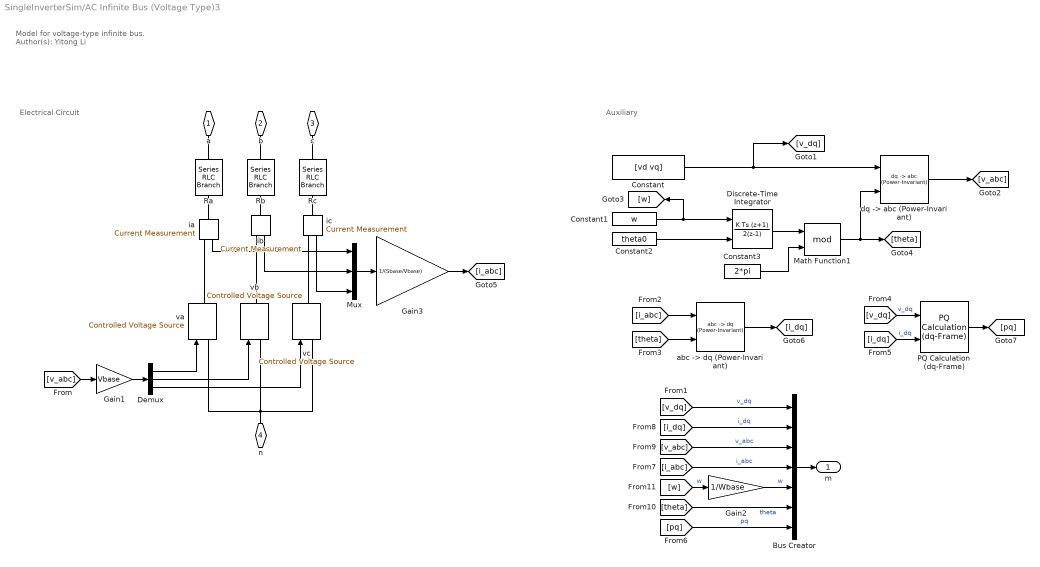
== system SingleInverterSim/AC Infinite Bus (Voltage Type)3 ==
  note: Model for voltage-type infinite bus.
      |
      | Author(s): Yitong Li
  note: Electrical Circuit
  note: Auxiliary
  Bus Creator : BusCreator  Inputs=7
  Constant : Constant  Value=[vd vq]
  Constant1 : Constant  Value=w
  Constant2 : Constant  Value=theta0
  Constant3 : Constant  Value=2*pi
  Demux : Demux  Outputs=3
  Discrete-Time Integrator : DiscreteIntegrator  IntegratorMethod=Integration: Trapezoidal  InitialConditionSource=external  SampleTime=-1  ICPrevOutput=DiscIntNeverNeededParam  ICPrevScaledInput=DiscIntNeverNeededParam
  Gain1 : Gain  Gain=Vbase
  Gain2 : Gain  Gain=1/Wbase
  Gain3 : Gain  Gain=1/(Sbase/Vbase)
  Math Function1 : Math  Operator=mod  SignedPower=on  SaturateOnIntegerOverflow=on
  Mux : Mux  Inputs=3
  PQ Calculation (dq-Frame) : SimplexPS/PQ Calculation (dq-Frame)  SystemSampleTime=-1  VariantActivationTime=update diagram  Latency=0  AutoFrameSizeCalculation=off
      settings: SourceProductName=Simplex Power Systems
  Ra : powerlib/Elements/Series RLC Branch  LConnTagsString=__new0  RConnTagsString=__new0  BranchType=R  Resistance=R  Inductance=1e-3  SetiL0=off  InitialCurrent=0  Capacitance=1e-6  Setx0=off  InitialVoltage=0  Measurements=None
  Rb : powerlib/Elements/Series RLC Branch  LConnTagsString=__new0  RConnTagsString=__new0  BranchType=R  Resistance=R  Inductance=1e-3  SetiL0=off  InitialCurrent=0  Capacitance=1e-6  Setx0=off  InitialVoltage=0  Measurements=None
  Rc : powerlib/Elements/Series RLC Branch  LConnTagsString=__new0  RConnTagsString=__new0  BranchType=R  Resistance=R  Inductance=1e-3  SetiL0=off  InitialCurrent=0  Capacitance=1e-6  Setx0=off  InitialVoltage=0  Measurements=None
  "abc -> dq (Power-Invariant)" : SimplexPS/abc -> dq (Power-Invariant)  SystemSampleTime=-1  VariantActivationTime=update diagram  Latency=0  AutoFrameSizeCalculation=off
      settings: SourceProductName=Simplex Power Systems
  "dq -> abc (Power-Invariant)" : SimplexPS/dq -> abc (Power-Invariant)  SystemSampleTime=-1  VariantActivationTime=update diagram  Latency=0  AutoFrameSizeCalculation=off
      settings: SourceProductName=Simplex Power Systems
  ia : powerlib/Measurements/Current Measurement  PhasorSimulation=off  OutputType=Complex  PSBequivalent=0
  ib : powerlib/Measurements/Current Measurement  PhasorSimulation=off  OutputType=Complex  PSBequivalent=0
  ic : powerlib/Measurements/Current Measurement  PhasorSimulation=off  OutputType=Complex  PSBequivalent=0
  va : powerlib/Electrical Sources/Controlled Voltage Source  Initialize=on  Source_Type=AC  Amplitude=0  Phase=0  Frequency=0  Measurements=None
  vb : powerlib/Electrical Sources/Controlled Voltage Source  Initialize=on  Source_Type=AC  Amplitude=0  Phase=0  Frequency=0  Measurements=None
  vc : powerlib/Electrical Sources/Controlled Voltage Source  Initialize=on  Source_Type=AC  Amplitude=0  Phase=0  Frequency=0  Measurements=None
  a : PMIOPort  Side=Left
  b : PMIOPort  Port=2  Side=Left
  c : PMIOPort  Port=3  Side=Left
  n : PMIOPort  Port=4  Side=Left
  m : Outport
  wires:
  [v_abc] -> Gain1/1
  Demux/1 -> va/1
  Demux/2 -> vb/1
  Demux/3 -> vc/1
  Math Function1/1 -> "dq -> abc (Power-Invariant)"/2, [theta]
  Constant2/1 -> Discrete-Time Integrator/2
  Constant1/1 -> Discrete-Time Integrator/1, [w]
  "dq -> abc (Power-Invariant)"/1 -> [v_abc]
  Constant3/1 -> Math Function1/2
  Constant/1 -> "dq -> abc (Power-Invariant)"/1, [v_dq]
  Discrete-Time Integrator/1 -> Math Function1/1
  [v_dq] -> Bus Creator/1  "v_dq"
  [i_abc] -> Bus Creator/4  "i_abc"
  [w] -> Gain2/1  "w"
  [v_abc] -> Bus Creator/3  "v_abc"
  Gain2/1 -> Bus Creator/5  "w"
  [i_dq] -> Bus Creator/2  "i_dq"
  Bus Creator/1 -> m/1
  [theta] -> Bus Creator/6  "theta"
  ia/1 -> Mux/1
  ib/1 -> Mux/2
  ic/1 -> Mux/3
  [i_abc] -> "abc -> dq (Power-Invariant)"/1
  [theta] -> "abc -> dq (Power-Invariant)"/2
  "abc -> dq (Power-Invariant)"/1 -> [i_dq]
  Gain1/1 -> Demux/1
  Mux/1 -> Gain3/1
  Gain3/1 -> [i_abc]
  [v_dq] -> PQ Calculation (dq-Frame)/1  "v_dq"
  [i_dq] -> PQ Calculation (dq-Frame)/2  "i_dq"
  PQ Calculation (dq-Frame)/1 -> [pq]
  [pq] -> Bus Creator/7  "pq"
  connections:
  vc/LConn1 -- n/RConn1 -- va/LConn1 -- vb/LConn1
  ia/RConn1 -- va/RConn1
  ib/RConn1 -- vb/RConn1
  ic/RConn1 -- vc/RConn1
  Ra/RConn1 -- ia/LConn1
  Ra/LConn1 -- a/RConn1
  ib/LConn1 -- Rb/RConn1
  Rb/LConn1 -- b/RConn1
  Rc/RConn1 -- ic/LConn1
  Rc/LConn1 -- c/RConn1

== system SingleInverterSim/AC Infinite Bus (Voltage Type)4 ==
  note: Model for voltage-type infinite bus.
      |
      | Author(s): Yitong Li
  note: Electrical Circuit
  note: Auxiliary
  Bus Creator : BusCreator  Inputs=7
  Constant : Constant  Value=[vd vq]
  Constant1 : Constant  Value=w
  Constant2 : Constant  Value=theta0
  Constant3 : Constant  Value=2*pi
  Demux : Demux  Outputs=3
  Discrete-Time Integrator : DiscreteIntegrator  IntegratorMethod=Integration: Trapezoidal  InitialConditionSource=external  SampleTime=-1  ICPrevOutput=DiscIntNeverNeededParam  ICPrevScaledInput=DiscIntNeverNeededParam
  Gain1 : Gain  Gain=Vbase
  Gain2 : Gain  Gain=1/Wbase
  Gain3 : Gain  Gain=1/(Sbase/Vbase)
  Math Function1 : Math  Operator=mod  SignedPower=on  SaturateOnIntegerOverflow=on
  Mux : Mux  Inputs=3
  PQ Calculation (dq-Frame) : SimplexPS/PQ Calculation (dq-Frame)  SystemSampleTime=-1  VariantActivationTime=update diagram  Latency=0  AutoFrameSizeCalculation=off
      settings: SourceProductName=Simplex Power Systems
  Ra : powerlib/Elements/Series RLC Branch  LConnTagsString=__new0  RConnTagsString=__new0  BranchType=R  Resistance=R  Inductance=1e-3  SetiL0=off  InitialCurrent=0  Capacitance=1e-6  Setx0=off  InitialVoltage=0  Measurements=None
  Rb : powerlib/Elements/Series RLC Branch  LConnTagsString=__new0  RConnTagsString=__new0  BranchType=R  Resistance=R  Inductance=1e-3  SetiL0=off  InitialCurrent=0  Capacitance=1e-6  Setx0=off  InitialVoltage=0  Measurements=None
  Rc : powerlib/Elements/Series RLC Branch  LConnTagsString=__new0  RConnTagsString=__new0  BranchType=R  Resistance=R  Inductance=1e-3  SetiL0=off  InitialCurrent=0  Capacitance=1e-6  Setx0=off  InitialVoltage=0  Measurements=None
  "abc -> dq (Power-Invariant)" : SimplexPS/abc -> dq (Power-Invariant)  SystemSampleTime=-1  VariantActivationTime=update diagram  Latency=0  AutoFrameSizeCalculation=off
      settings: SourceProductName=Simplex Power Systems
  "dq -> abc (Power-Invariant)" : SimplexPS/dq -> abc (Power-Invariant)  SystemSampleTime=-1  VariantActivationTime=update diagram  Latency=0  AutoFrameSizeCalculation=off
      settings: SourceProductName=Simplex Power Systems
  ia : powerlib/Measurements/Current Measurement  PhasorSimulation=off  OutputType=Complex  PSBequivalent=0
  ib : powerlib/Measurements/Current Measurement  PhasorSimulation=off  OutputType=Complex  PSBequivalent=0
  ic : powerlib/Measurements/Current Measurement  PhasorSimulation=off  OutputType=Complex  PSBequivalent=0
  va : powerlib/Electrical Sources/Controlled Voltage Source  Initialize=on  Source_Type=AC  Amplitude=0  Phase=0  Frequency=0  Measurements=None
  vb : powerlib/Electrical Sources/Controlled Voltage Source  Initialize=on  Source_Type=AC  Amplitude=0  Phase=0  Frequency=0  Measurements=None
  vc : powerlib/Electrical Sources/Controlled Voltage Source  Initialize=on  Source_Type=AC  Amplitude=0  Phase=0  Frequency=0  Measurements=None
  a : PMIOPort  Side=Left
  b : PMIOPort  Port=2  Side=Left
  c : PMIOPort  Port=3  Side=Left
  n : PMIOPort  Port=4  Side=Left
  m : Outport
  wires:
  [v_abc] -> Gain1/1
  Demux/1 -> va/1
  Demux/2 -> vb/1
  Demux/3 -> vc/1
  Math Function1/1 -> "dq -> abc (Power-Invariant)"/2, [theta]
  Constant2/1 -> Discrete-Time Integrator/2
  Constant1/1 -> Discrete-Time Integrator/1, [w]
  "dq -> abc (Power-Invariant)"/1 -> [v_abc]
  Constant3/1 -> Math Function1/2
  Constant/1 -> "dq -> abc (Power-Invariant)"/1, [v_dq]
  Discrete-Time Integrator/1 -> Math Function1/1
  [v_dq] -> Bus Creator/1  "v_dq"
  [i_abc] -> Bus Creator/4  "i_abc"
  [w] -> Gain2/1  "w"
  [v_abc] -> Bus Creator/3  "v_abc"
  Gain2/1 -> Bus Creator/5  "w"
  [i_dq] -> Bus Creator/2  "i_dq"
  Bus Creator/1 -> m/1
  [theta] -> Bus Creator/6  "theta"
  ia/1 -> Mux/1
  ib/1 -> Mux/2
  ic/1 -> Mux/3
  [i_abc] -> "abc -> dq (Power-Invariant)"/1
  [theta] -> "abc -> dq (Power-Invariant)"/2
  "abc -> dq (Power-Invariant)"/1 -> [i_dq]
  Gain1/1 -> Demux/1
  Mux/1 -> Gain3/1
  Gain3/1 -> [i_abc]
  [v_dq] -> PQ Calculation (dq-Frame)/1  "v_dq"
  [i_dq] -> PQ Calculation (dq-Frame)/2  "i_dq"
  PQ Calculation (dq-Frame)/1 -> [pq]
  [pq] -> Bus Creator/7  "pq"
  connections:
  vc/LConn1 -- n/RConn1 -- va/LConn1 -- vb/LConn1
  ia/RConn1 -- va/RConn1
  ib/RConn1 -- vb/RConn1
  ic/RConn1 -- vc/RConn1
  Ra/RConn1 -- ia/LConn1
  Ra/LConn1 -- a/RConn1
  ib/LConn1 -- Rb/RConn1
  Rb/LConn1 -- b/RConn1
  Rc/RConn1 -- ic/LConn1
  Rc/LConn1 -- c/RConn1
